simulink model "RoboticsCW1"  (R2022b)
settings: Solver=VariableStepAuto  StartTime=0.0  StopTime=10.0  RelTol=1e-3
settings Model: Creator=nikee  LastModifiedBy=nikee

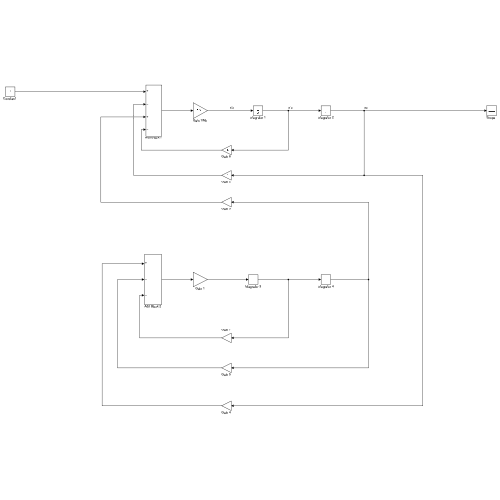
[thumbnail: Simulink's stored preview of the top-level diagram]
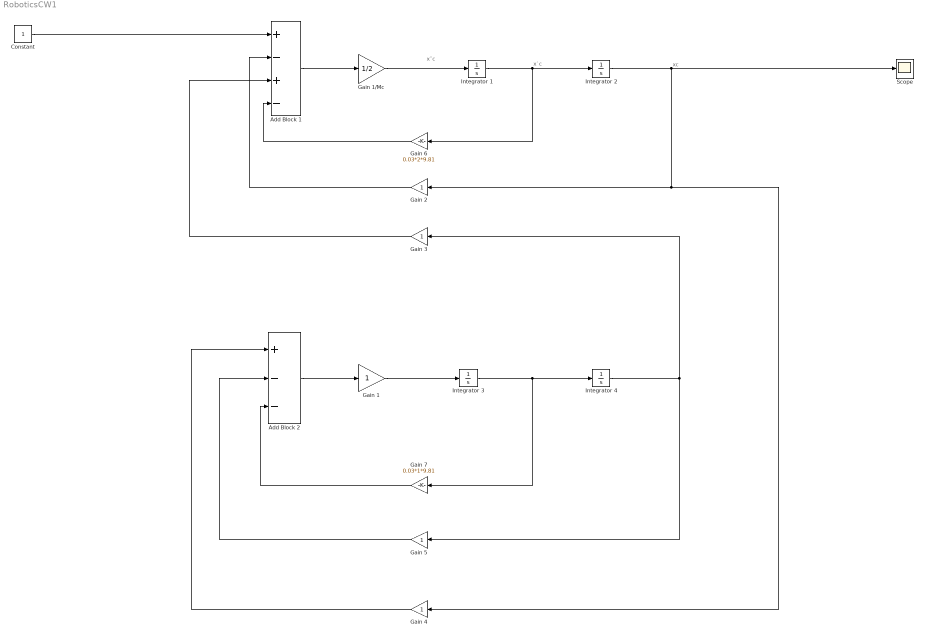
== system RoboticsCW1 ==
  note: xc
  note: x˙c
  note: x¨c
  Add Block 1 : Sum  Inputs=+-+-
  Add Block 2 : Sum  Inputs=+--
  "Constant " : Constant
  Gain {1,3..5} (4 alike) : Gain
  Gain 1/Mc : Gain  Gain=1/2
  Gain 2 : Gain  ParamMax=[2]
  Gain 6 : Gain  Gain=0.03*2*9.81  ParamMax=[2]
  Gain 7 : Gain  Gain=0.03*1*9.81
  Integrator {1..4} (4 alike) : Integrator
  "Scope " : Scope
  wires:
  Gain 6/1 -> Add Block 1/4
  "Constant "/1 -> Add Block 1/1
  Gain 3/1 -> Add Block 1/3
  Gain 5/1 -> Add Block 2/2
  Gain 7/1 -> Add Block 2/3
  Integrator 2/1 -> Gain 4/1, Gain 2/1, "Scope "/1
  Gain 4/1 -> Add Block 2/1
  Add Block 1/1 -> Gain 1/Mc/1
  Integrator 1/1 -> Gain 6/1, Integrator 2/1
  Integrator 4/1 -> Gain 5/1, Gain 3/1
  Gain 2/1 -> Add Block 1/2
  Add Block 2/1 -> Gain 1/1
  Integrator 3/1 -> Gain 7/1, Integrator 4/1
  Gain 1/1 -> Integrator 3/1
  Gain 1/Mc/1 -> Integrator 1/1
